simulink model "navigation"  (R2020a)
settings: Solver=VariableStepAuto  StartTime=0.0  StopTime=inf  RelTol=1e-3
model workspace (MAT data in the model file):
  Logfile_Data_Object = robotics.ros.BagSelection
  Logfile_Data_Object.FilePath = '/home/john/github/Thesis-/Control Algorithms/Navigation_Stack/Experiment_6_Plots/2022-08-07-23-07-18.bag'
  Logfile_Data_Object.StartTime = 1659877638.2
  Logfile_Data_Object.EndTime = 1659877673.93
  Logfile_Data_Object.NumMessages = 1808
  Logfile_Data_Object.AvailableTopics = table
  Logfile_Data_Object.AvailableTopics.data{1} = [36; 36; 714; 1022]
  Logfile_Data_Object.AvailableTopics.data{2} = categorical
  Logfile_Data_Object.AvailableTopics.data{2}.categoryNames = {'nav_msgs/Odometry'; 'std_msgs/Float32'; 'std_msgs/Float32MultiArray'}
  Logfile_Data_Object.AvailableTopics.data{2}.codes = [2; 2; 1; 3]
  Logfile_Data_Object.AvailableTopics.data{3}{1} = ''
  Logfile_Data_Object.AvailableTopics.data{3}{2} = ''
  Logfile_Data_Object.AvailableTopics.data{3}{3} = '  uint32 Seq
    |   Time Stamp
    |   char FrameId
    | char ChildFrameId
    | geometry_msgs/PoseWithCovariance Pose
    |   geometry_msgs/Pose Pose
    |     geometry_msgs/Point Position
    |       double X
    |       double Y
    |       double Z
    |     geometry_msgs/Quaternion Orientation
    |       double X
    |       double Y
    |       double Z
    |       double W
    |   double[36] Covariance
    | geometry_msgs/TwistWithCovariance Twist
    |   geometry_msgs/Twist Twist
    |     geometry_msgs/Vector3 Linear
    |       double X
    |       double Y
    |       double Z
    |     geometry_msgs/Vector3 Angular
    |       double X
    |       double Y
    |       double Z
    |   double[36] Covariance
    | '
  Logfile_Data_Object.AvailableTopics.data{3}{4} = '  std_msgs/MultiArrayDimension[] Dim
    |     char Label
    |     uint32 Size
    |     uint32 Stride
    |   uint32 DataOffset
    | single[] Data
    | '
  Logfile_Data_Object.AvailableTopics.ndims = 2
  Logfile_Data_Object.AvailableTopics.nrows = 4
  Logfile_Data_Object.AvailableTopics.rownames = {'/amr/status/current'; '/amr/status/voltage'; '/slamware_ros_sdk_server_node/odom'; '/zlac8015d/encoder'}
  Logfile_Data_Object.AvailableTopics.nvars = 3
  Logfile_Data_Object.AvailableTopics.varnames = {'NumMessages', 'MessageType', 'MessageDefinition'}
  Logfile_Data_Object.AvailableTopics.props.useVariableNamesOriginal = 0
  Logfile_Data_Object.AvailableTopics.props.useDimensionNamesOriginal = 0
  Logfile_Data_Object.AvailableTopics.props.CustomProps = struct()
  Logfile_Data_Object.AvailableTopics.props.VariableCustomProps = struct()
  Logfile_Data_Object.AvailableTopics.props.versionSavedFrom = 4
  Logfile_Data_Object.AvailableTopics.props.minCompatibleVersion = 1
  Logfile_Data_Object.AvailableTopics.props.incompatibilityMsg = ''
  Logfile_Data_Object.AvailableTopics.props.VersionSavedFrom = 4
  Logfile_Data_Object.AvailableTopics.props.Description = ''
  Logfile_Data_Object.AvailableTopics.props.VariableNamesOriginal = {}
  Logfile_Data_Object.AvailableTopics.props.DimensionNames = {'Row', 'Variables'}
  Logfile_Data_Object.AvailableTopics.props.DimensionNamesOriginal = {}
  Logfile_Data_Object.AvailableTopics.props.UserData = []
  Logfile_Data_Object.AvailableTopics.props.VariableDescriptions = {}
  Logfile_Data_Object.AvailableTopics.props.VariableUnits = {}
  Logfile_Data_Object.AvailableTopics.props.VariableContinuity = {}
  Logfile_Data_Object.MessageList = table
  Logfile_Data_Object.MessageList.data{1} = [1659877638.2 1659877638.22 1659877638.24 1659877638.25 1659877638.29 1659877638.29 1659877638.32 1659877638.34 1659877638.35 1659877638.38 1659877638.39 1659877638.41 ... (1808 elements, 1808x1)]
  Logfile_Data_Object.MessageList.data{2} = categorical
  Logfile_Data_Object.MessageList.data{2}.categoryNames = {'/amr/status/current'; '/amr/status/voltage'; '/slamware_ros_sdk_server_node/odom'; '/zlac8015d/encoder'}
  Logfile_Data_Object.MessageList.data{2}.codes = [3 4 3 4 4 3 4 3 4 4 3 4 ... (1808 elements, 1808x1)]
  Logfile_Data_Object.MessageList.data{3} = categorical
  Logfile_Data_Object.MessageList.data{3}.categoryNames = {'std_msgs/Float32'; 'nav_msgs/Odometry'; 'std_msgs/Float32MultiArray'}
  Logfile_Data_Object.MessageList.data{3}.codes = [2 3 2 3 3 2 3 2 3 3 2 3 ... (1808 elements, 1808x1)]
  Logfile_Data_Object.MessageList.data{4} = [7710 10178 10256 11007 11085 11163 11914 11992 12743 12821 12899 13650 ... (1808 elements, 1808x1)]
  Logfile_Data_Object.MessageList.ndims = 2
  Logfile_Data_Object.MessageList.nrows = 1808
  Logfile_Data_Object.MessageList.nvars = 4
  Logfile_Data_Object.MessageList.varnames = {'Time', 'Topic', 'MessageType', 'FileOffset'}
  Logfile_Data_Object.MessageList.props.useVariableNamesOriginal = 0
  Logfile_Data_Object.MessageList.props.useDimensionNamesOriginal = 0
  Logfile_Data_Object.MessageList.props.CustomProps = struct()
  Logfile_Data_Object.MessageList.props.VariableCustomProps = struct()
  Logfile_Data_Object.MessageList.props.versionSavedFrom = 4
  Logfile_Data_Object.MessageList.props.minCompatibleVersion = 1
  Logfile_Data_Object.MessageList.props.incompatibilityMsg = ''
  Logfile_Data_Object.MessageList.props.VersionSavedFrom = 4
  Logfile_Data_Object.MessageList.props.Description = ''
  Logfile_Data_Object.MessageList.props.VariableNamesOriginal = {}
  Logfile_Data_Object.MessageList.props.DimensionNames = {'Row', 'Variables'}
  Logfile_Data_Object.MessageList.props.DimensionNamesOriginal = {}
  Logfile_Data_Object.MessageList.props.UserData = []
  Logfile_Data_Object.MessageList.props.VariableDescriptions = {}
  Logfile_Data_Object.MessageList.props.VariableUnits = {}
  Logfile_Data_Object.MessageList.props.VariableContinuity = {}
  Logfile_Data_Object.TopicTypeMap = containers.Map
  Logfile_Data_Object.TopicTypeMap.serialization.keys = {'/amr/status/current', '/amr/status/voltage', '/slamware_ros_sdk_server_node/odom', '/zlac8015d/encoder'}
  Logfile_Data_Object.TopicTypeMap.serialization.values = {'std_msgs/Float32', 'std_msgs/Float32', 'nav_msgs/Odometry', 'std_msgs/Float32MultiArray'}
  Logfile_Data_Object.TopicTypeMap.serialization.uniformity = 1
  Logfile_Data_Object.TopicTypeMap.serialization.keyType = 'char'
  Logfile_Data_Object.TopicTypeMap.serialization.valueType = 'char'
  Logfile_Data_Object.TopicDefinitionMap = containers.Map
  Logfile_Data_Object.TopicDefinitionMap.serialization.keys = {'/amr/status/current', '/amr/status/voltage', '/slamware_ros_sdk_server_node/odom', '/zlac8015d/encoder'}
  Logfile_Data_Object.TopicDefinitionMap.serialization.values{1} = ''
  Logfile_Data_Object.TopicDefinitionMap.serialization.values{2} = ''
  Logfile_Data_Object.TopicDefinitionMap.serialization.values{3} = '  uint32 Seq
    |   Time Stamp
    |   char FrameId
    | char ChildFrameId
    | geometry_msgs/PoseWithCovariance Pose
    |   geometry_msgs/Pose Pose
    |     geometry_msgs/Point Position
    |       double X
    |       double Y
    |       double Z
    |     geometry_msgs/Quaternion Orientation
    |       double X
    |       double Y
    |       double Z
    |       double W
    |   double[36] Covariance
    | geometry_msgs/TwistWithCovariance Twist
    |   geometry_msgs/Twist Twist
    |     geometry_msgs/Vector3 Linear
    |       double X
    |       double Y
    |       double Z
    |     geometry_msgs/Vector3 Angular
    |       double X
    |       double Y
    |       double Z
    |   double[36] Covariance
    | '
  Logfile_Data_Object.TopicDefinitionMap.serialization.values{4} = '  std_msgs/MultiArrayDimension[] Dim
    |     char Label
    |     uint32 Size
    |     uint32 Stride
    |   uint32 DataOffset
    | single[] Data
    | '
  Logfile_Data_Object.TopicDefinitionMap.serialization.uniformity = 1
  Logfile_Data_Object.TopicDefinitionMap.serialization.keyType = 'char'
  Logfile_Data_Object.TopicDefinitionMap.serialization.valueType = 'char'
  Logfile_Data_Object.Parser = robotics.ros.internal.tf.TransformationTreeParser
  Logfile_Path = '/home/john/github/Thesis-/Control Algorithms/Navigation_Stack/Experiment_6_Plots/2022-08-07-23-07-18.bag'
  Logfile_Playback_Duration = nan
  Logfile_Playback_Offset = nan
values from neighbouring files (symbols this model uses):
  C = [1 0 0 ... (first row only)    [start.m]
  D = [0 0 ... (first row only)    [start.m]
  encoderSampleRate = 10    [start.m]
  firstGoal = [1.5,1.5]    [start.m]
  initialInput = [0; 0]    [start.m]
  initialPose = [0, 0, 0]    [start.m]
  L2RTransform = [cos(L2Rtheta), -sin(L2Rtheta), L2Rx ... (first row only)    [start.m]    (also in test.m = [0.0073926; -0.32076; (3/2)*pi])
  LIVE_MODE = 1    [start.m]
  pose = [0;0;0]    [test.m]
  R = diag(RVar*ones(yNum,1))    [start.m]
  secondGoal = [0.5,0.5]    [start.m]
  timeStep = 0.1    [start.m]
  W2LOTransform = [cos(W2LOtheta), -sin(W2LOtheta), W2LOx ... (first row only)    [start.m]
  W2ORTransform = [cos(W2ORtheta), -sin(W2ORtheta), W2ORx ... (first row only)    [start.m]
  wheelBase = 0.4464    [start.m]
  wheelRadius = 0.1715/2    (= 0.08575)    [start.m]
undefined symbols (not defined in the file or in its folder): Angular, Discrete, goalLoc, startLoc, Time
libraries: robotlib x9, simulink x5, robotmobilelib x3, robotalgslib x3, ctrlSharedLib x1
settings Model: EnablePacing=on  Creator=johni  LastModifiedBy=john

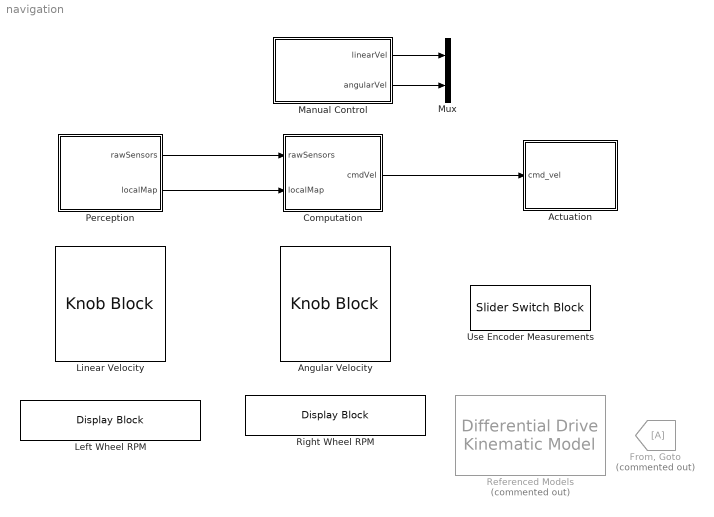
== system navigation ==
  Actuation : Subsystem
  Angular Velocity : KnobBlock  ScaleMin=-1  ScaleMax=1
  Computation : Subsystem
  "From, Goto" : Goto  Commented=on
  Left Wheel RPM : DisplayBlock  LabelPosition=Hide  Format=short  Transparency=1
  Linear Velocity : KnobBlock  ScaleMin=-0.5  ScaleMax=0.5
  Manual Control : Subsystem
  Mux : Mux  Inputs=2
  Perception : Subsystem
  Referenced Models : robotmobilelib/Differential Drive Kinematic Model  Commented=on  VehicleInputs=Wheel Speeds  WheelRadius=0.05  WheelSpeedRange=[-inf inf]  TrackWidth=0.2  InitialState=[0; 0; 0]  SimulateUsing=Interpreted execution
      settings: SourceProductBaseCode=RO
  Right Wheel RPM : DisplayBlock  LabelPosition=Hide  Format=short  Transparency=1
  Use Encoder Measurements : SliderSwitchBlock
      settings: Values={{'Off', 'On'}, [0 1]}
  wires:
  Perception/1(rawSensors) -> Computation/1(rawSensors)
  Perception/2(localMap) -> Computation/2(localMap)
  Manual Control/2(angularVel) -> Mux/2
  Manual Control/1(linearVel) -> Mux/1
  Computation/1(cmdVel) -> Actuation/1(cmd_vel)

== system navigation/Actuation ==
  cmd_vel : Inport
  Actuator : Subsystem
  Demux : Demux  Outputs=2
  Forward Kinematics : Subsystem
  Subsystem : Subsystem  Commented=on
  wires:
  cmd_vel/1 -> Demux/1
  Forward Kinematics/1(leftRpmOut) -> Subsystem/1(leftRPM), Actuator/1(leftRPM)
  Forward Kinematics/2(rightRpmOut) -> Subsystem/2(rightRPM), Actuator/2(rightRPM)
  Demux/2 -> Forward Kinematics/2(w_in)
  Demux/1 -> Forward Kinematics/1(v_in)

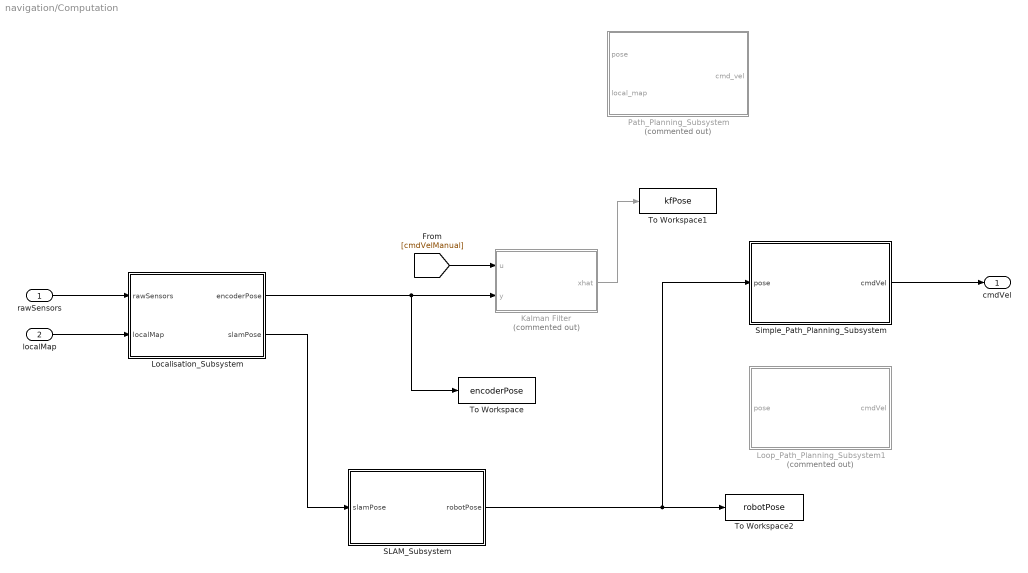
== system navigation/Computation ==
  rawSensors : Inport
  localMap : Inport  Port=2
  Kalman Filter : Subsystem  Commented=on
  Localisation_Subsystem : Subsystem
  Loop_Path_Planning_Subsystem1 : Subsystem  Commented=on
  Path_Planning_Subsystem : Subsystem  Commented=on
  SLAM_Subsystem : Subsystem
  Simple_Path_Planning_Subsystem : Subsystem
  To Workspace : ToWorkspace  VariableName=encoderPose  SaveFormat=Timeseries  SampleTime=-1
  To Workspace1 : ToWorkspace  VariableName=kfPose  SaveFormat=Timeseries  SampleTime=-1
  To Workspace2 : ToWorkspace  VariableName=robotPose  SaveFormat=Timeseries  SampleTime=-1
  cmdVel : Outport
  wires:
  rawSensors/1 -> Localisation_Subsystem/1(rawSensors)
  localMap/1 -> Localisation_Subsystem/2(localMap)
  Localisation_Subsystem/1(encoderPose) -> To Workspace/1, Kalman Filter/2(y)
  SLAM_Subsystem/1(robotPose) -> Simple_Path_Planning_Subsystem/1(pose), To Workspace2/1
  Kalman Filter/1(xhat) -> To Workspace1/1
  [cmdVelManual] -> Kalman Filter/1(u)
  Localisation_Subsystem/2(slamPose) -> SLAM_Subsystem/1(slamPose)
  Simple_Path_Planning_Subsystem/1(cmdVel) -> cmdVel/1

== system navigation/Manual Control ==
  Constant1 : Constant  Value=-0.0004086893464075869
  Constant2 : Constant  Value=0.01208821805826843
  linearVel : Outport
  angularVel : Outport  Port=2
  wires:
  Constant2/1 -> angularVel/1
  Constant1/1 -> linearVel/1

== system navigation/Perception ==
  Encoder_Subsystem : Subsystem
  IMU_Subsystem : Subsystem  Commented=on
  Lidar_Subsystem : Subsystem
  Mux2 : Mux  Inputs=6
  rawSensors : Outport
  localMap : Outport  Port=2
  wires:
  Mux2/1 -> rawSensors/1
  Lidar_Subsystem/3(localMap) -> localMap/1
  IMU_Subsystem/2(linearAcceleration) -> Mux2/4
  IMU_Subsystem/1(angularVelocity) -> Mux2/3
  Lidar_Subsystem/2(slamPose) -> Mux2/6
  Lidar_Subsystem/1(laserScan) -> Mux2/5
  Encoder_Subsystem/2(rightSpeed) -> Mux2/2
  Encoder_Subsystem/1(leftSpeed) -> Mux2/1

== system navigation/Actuation/Actuator ==
  leftRPM : Inport
  rightRPM : Inport  Port=2
  Blank Message : robotlib/Blank Message  messageClass=Message  entityType=geometry_msgs/Twist  messageType=geometry_msgs/Twist  SampleTime=inf
  Bus Assignment : BusAssignment  AssignedSignals=Angular.X,Angular.Y
  Publish : robotlib/Publish  topicSource=Select from ROS network  topic=/zlac8015d/rpm  messageType=geometry_msgs/Twist  messageQueueLength=1
  wires:
  Bus Assignment/1 -> Publish/1
  Blank Message/1 -> Bus Assignment/1
  rightRPM/1 -> Bus Assignment/3
  leftRPM/1 -> Bus Assignment/2

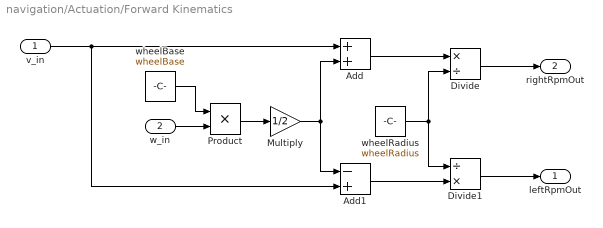
== system navigation/Actuation/Forward Kinematics ==
  v_in : Inport
  w_in : Inport  Port=2
  Add : Sum
  Add1 : Sum  Inputs=-+
  Divide : Product  Inputs=*/
  Divide1 : Product  Inputs=/*
  Multiply : Gain  Gain=1/2
  Product : Product
  wheelBase : Constant  Value=wheelBase
  wheelRadius : Constant  Value=wheelRadius
  leftRpmOut : Outport
  rightRpmOut : Outport  Port=2
  wires:
  v_in/1 -> Add1/2, Add/1
  w_in/1 -> Product/2
  wheelBase/1 -> Product/1
  Product/1 -> Multiply/1
  Multiply/1 -> Add/2, Add1/1
  Add1/1 -> Divide1/2
  Add/1 -> Divide/1
  wheelRadius/1 -> Divide1/1, Divide/2
  Divide1/1 -> leftRpmOut/1
  Divide/1 -> rightRpmOut/1

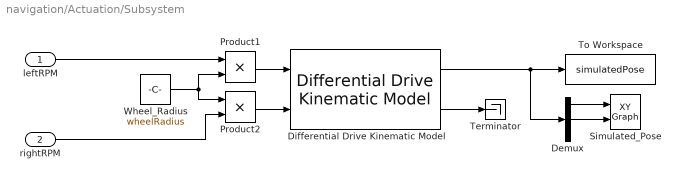
== system navigation/Actuation/Subsystem ==
  leftRPM : Inport
  rightRPM : Inport  Port=2
  Demux : Demux  Outputs=3
  Differential Drive Kinematic Model : robotmobilelib/Differential Drive Kinematic Model  VehicleInputs=Wheel Speeds  WheelRadius=wheelRadius  WheelSpeedRange=[-inf inf]  TrackWidth=wheelBase  InitialState=initialPose  SimulateUsing=Interpreted execution
      settings: SourceProductBaseCode=RO
  Product1 : Product
  Product2 : Product
  Simulated_Pose : simulink/Sinks/XY Graph  xmin=-1.5  xmax=1.5  ymin=-1.5  ymax=1.5  st=-1
  Terminator : Terminator
  To Workspace : ToWorkspace  VariableName=simulatedPose  SaveFormat=Timeseries  SampleTime=-1
  Wheel_Radius : Constant  Value=wheelRadius
  wires:
  Differential Drive Kinematic Model/1 -> Demux/1, To Workspace/1
  Differential Drive Kinematic Model/2 -> Terminator/1
  Demux/2 -> Simulated_Pose/2
  Demux/1 -> Simulated_Pose/1
  Product2/1 -> Differential Drive Kinematic Model/2
  Wheel_Radius/1 -> Product2/1, Product1/2
  leftRPM/1 -> Product1/1
  rightRPM/1 -> Product2/2
  Product1/1 -> Differential Drive Kinematic Model/1

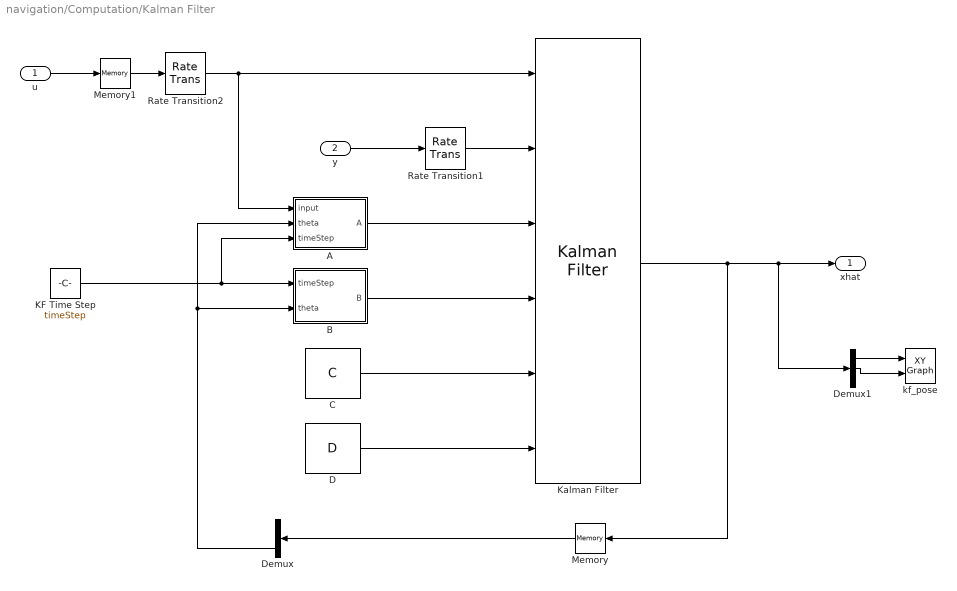
== system navigation/Computation/Kalman Filter ==
  u : Inport
  y : Inport  Port=2
  A : MATLAB Function  TreatAsAtomicUnit=on
  B : MATLAB Function  TreatAsAtomicUnit=on
  C : Constant  Value=C
  D : Constant  Value=D
  Demux : Demux  Outputs=3
  Demux1 : Demux  Outputs=3
  KF Time Step : Constant  Value=timeStep
  Kalman Filter : ctrlSharedLib/Kalman Filter  TimeDomain=Discrete-Time  UseCurrentEstimator=on  ModelSource=Input port  ModelSourceVariable=ss(0.95,1,1,0,1)  A=[1 0 0; 0 1 0; 0 0 1;]  B=[cos(pose(1,3))*timeStep, 0; sin(pose(1,3))*timeStep, 0; 0 timeStep;]  C=[1 0 0; 0 1 0; 0 0 1;]  D=[0,0; 0,0; 0,0;]  NumberOfStates=xNum  NumberOfInputs=uNum  NumberOfOutputs=yNum  InitialEstimateSource=Dialog  X0=initialPose  P0=initialErrorCovariance  UseK=off  UseGH=off  NumberOfProcessNoiseInputs=1  G=1  TimeInvariantG=on  H=0  TimeInvariantH=on  Q=Q  TimeInvariantQ=on  R=R  TimeInvariantR=on  N=0  TimeInvariantN=on  AddInputPort=on  AddEnablePort=off  OutputEstimatedY=off  OutputP=off  Ts=timeStep
  Memory : Memory  InitialCondition=initialPose  InheritSampleTime=on
  Memory1 : Memory  InitialCondition=initialInput  InheritSampleTime=on
  Rate Transition1 : RateTransition  OutPortSampleTime=timeStep
  Rate Transition2 : RateTransition  OutPortSampleTime=timeStep
  kf_pose : simulink/Sinks/XY Graph  xmin=-3  xmax=3  ymin=-3  ymax=3  st=-1
  xhat : Outport
  wires:
  Kalman Filter/1 -> Demux1/1, xhat/1, Memory/1
  u/1 -> Memory1/1
  A/1(A) -> Kalman Filter/3
  C/1 -> Kalman Filter/5
  D/1 -> Kalman Filter/6
  Demux/3 -> A/2(theta), B/2(theta)
  B/1(B) -> Kalman Filter/4
  Memory/1 -> Demux/1
  KF Time Step/1 -> B/1(timeStep), A/3(timeStep)
  y/1 -> Rate Transition1/1
  Rate Transition1/1 -> Kalman Filter/2
  Memory1/1 -> Rate Transition2/1
  Demux1/1 -> kf_pose/1
  Demux1/2 -> kf_pose/2
  Rate Transition2/1 -> A/1(input), Kalman Filter/1

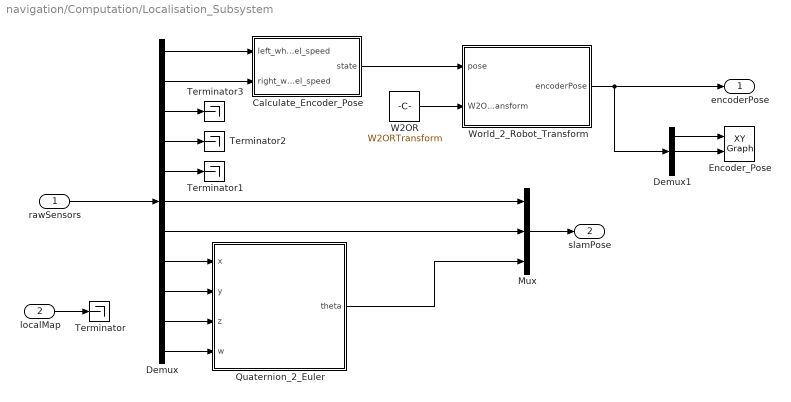
== system navigation/Computation/Localisation_Subsystem ==
  rawSensors : Inport
  localMap : Inport  Port=2
  Calculate_Encoder_Pose : Subsystem
  Demux : Demux  Outputs=11
  Demux1 : Demux  Outputs=3
  Encoder_Pose : simulink/Sinks/XY Graph  xmin=-1.5  xmax=1.5  ymin=-1.5  ymax=1.5  st=-1
  Mux : Mux  Inputs=3
  Quaternion_2_Euler : MATLAB Function  TreatAsAtomicUnit=on
  Terminator{,1..3} (4 alike) : Terminator
  W2OR : Constant  Value=W2ORTransform
  World_2_Robot_Transform : MATLAB Function  TreatAsAtomicUnit=on
  encoderPose : Outport
  slamPose : Outport  Port=2
  wires:
  rawSensors/1 -> Demux/1
  localMap/1 -> Terminator/1
  Demux/1 -> Calculate_Encoder_Pose/1(left_wheel_speed)
  Demux/2 -> Calculate_Encoder_Pose/2(right_wheel_speed)
  Demux/3 -> Terminator3/1
  Demux1/1 -> Encoder_Pose/1
  Demux1/2 -> Encoder_Pose/2
  Demux/4 -> Terminator2/1
  Demux/7 -> Mux/2
  Demux/6 -> Mux/1
  Demux/5 -> Terminator1/1
  Mux/1 -> slamPose/1
  Calculate_Encoder_Pose/1(state) -> World_2_Robot_Transform/1(pose)
  World_2_Robot_Transform/1(encoderPose) -> encoderPose/1, Demux1/1
  W2OR/1 -> World_2_Robot_Transform/2(W2ORTransform)
  Demux/8 -> Quaternion_2_Euler/1(x)
  Demux/9 -> Quaternion_2_Euler/2(y)
  Demux/10 -> Quaternion_2_Euler/3(z)
  Demux/11 -> Quaternion_2_Euler/4(w)
  Quaternion_2_Euler/1(theta) -> Mux/3

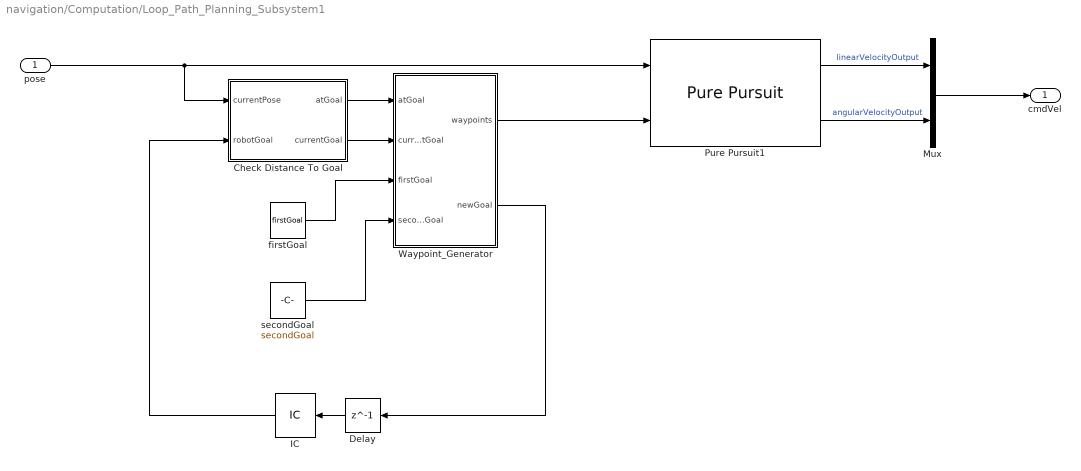
== system navigation/Computation/Loop_Path_Planning_Subsystem1 ==
  pose : Inport
  Check Distance To Goal : Subsystem
  Delay : Delay  DelayLength=1  InitialCondition=0
  IC : InitialCondition  Value=firstGoal
  Mux : Mux  Inputs=2
  Pure Pursuit1 : robotalgslib/Pure Pursuit  DesiredLinearVelocity=0.5  MaxAngularVelocity=1  LookaheadDistance=0.1  TargetDirPort=off  SimulateUsing=Code generation
  Waypoint_Generator : MATLAB Function  TreatAsAtomicUnit=on
  firstGoal : Constant  Value=firstGoal  VectorParams1D=off
  secondGoal : Constant  Value=secondGoal  VectorParams1D=off
  cmdVel : Outport
  wires:
  Mux/1 -> cmdVel/1
  pose/1 -> Check Distance To Goal/1(currentPose), Pure Pursuit1/1
  Pure Pursuit1/2 -> Mux/2  "angularVelocityOutput"
  Pure Pursuit1/1 -> Mux/1  "linearVelocityOutput"
  Check Distance To Goal/1(atGoal) -> Waypoint_Generator/1(atGoal)
  Check Distance To Goal/2(currentGoal) -> Waypoint_Generator/2(currentGoal)
  Waypoint_Generator/1(waypoints) -> Pure Pursuit1/2
  firstGoal/1 -> Waypoint_Generator/3(firstGoal)
  secondGoal/1 -> Waypoint_Generator/4(secondGoal)
  Waypoint_Generator/2(newGoal) -> Delay/1
  Delay/1 -> IC/1
  IC/1 -> Check Distance To Goal/2(robotGoal)

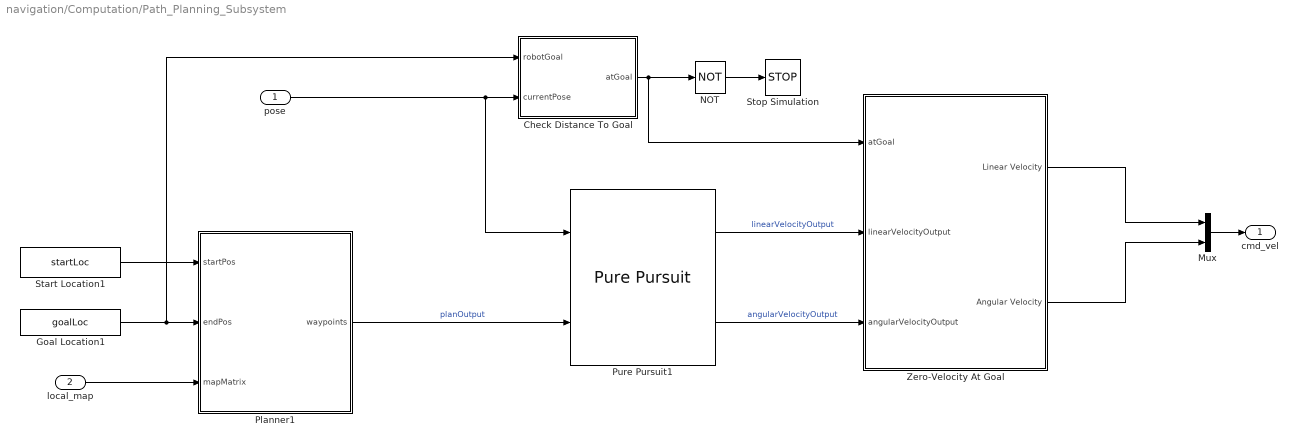
== system navigation/Computation/Path_Planning_Subsystem ==
  pose : Inport
  local_map : Inport  Port=2
  Check Distance To Goal : Subsystem
  Goal Location1 : Constant  Value=goalLoc
  Mux : Mux  Inputs=2
  NOT : Logic  Operator=NOT  IconShape=distinctive  AllPortsSameDT=off  OutDataTypeStr=boolean
  Planner1 : MATLAB Function  TreatAsAtomicUnit=on
  Pure Pursuit1 : robotalgslib/Pure Pursuit  DesiredLinearVelocity=0.1  MaxAngularVelocity=1.0  LookaheadDistance=0.5  TargetDirPort=off  SimulateUsing=Code generation
  Start Location1 : Constant  Value=startLoc
  Stop Simulation : Stop
  Zero-Velocity At Goal : Subsystem
  cmd_vel : Outport
  wires:
  local_map/1 -> Planner1/3(mapMatrix)
  Pure Pursuit1/2 -> Zero-Velocity At Goal/3(angularVelocityOutput)  "angularVelocityOutput"
  Pure Pursuit1/1 -> Zero-Velocity At Goal/2(linearVelocityOutput)  "linearVelocityOutput"
  Planner1/1(waypoints) -> Pure Pursuit1/2  "planOutput"
  NOT/1 -> Stop Simulation/1
  Start Location1/1 -> Planner1/1(startPos)
  Check Distance To Goal/1(atGoal) -> Zero-Velocity At Goal/1(atGoal), NOT/1
  Goal Location1/1 -> Check Distance To Goal/1(robotGoal), Planner1/2(endPos)
  pose/1 -> Pure Pursuit1/1, Check Distance To Goal/2(currentPose)
  Mux/1 -> cmd_vel/1
  Zero-Velocity At Goal/1(Linear Velocity) -> Mux/1
  Zero-Velocity At Goal/2(Angular Velocity) -> Mux/2

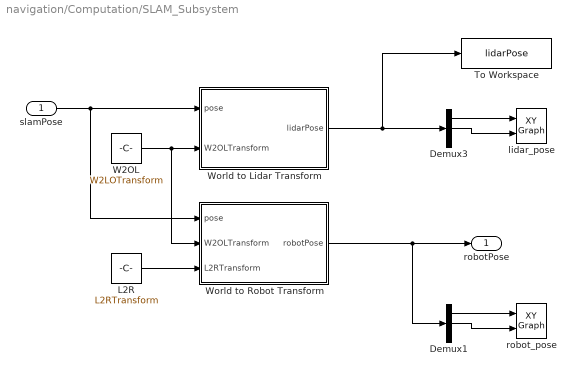
== system navigation/Computation/SLAM_Subsystem ==
  slamPose : Inport
  Demux1 : Demux  Outputs=3
  Demux3 : Demux  Outputs=3
  L2R : Constant  Value=L2RTransform
  To Workspace : ToWorkspace  VariableName=lidarPose  SaveFormat=Timeseries  SampleTime=-1
  W2OL : Constant  Value=W2LOTransform
  World to Lidar Transform : MATLAB Function  TreatAsAtomicUnit=on
  World to Robot Transform : MATLAB Function  TreatAsAtomicUnit=on
  lidar_pose : simulink/Sinks/XY Graph  xmin=0  xmax=3  ymin=0  ymax=3  st=-1
  robot_pose : simulink/Sinks/XY Graph  xmin=0  xmax=3  ymin=0  ymax=3  st=-1
  robotPose : Outport
  wires:
  Demux1/2 -> robot_pose/2
  Demux1/1 -> robot_pose/1
  slamPose/1 -> World to Robot Transform/1(pose), World to Lidar Transform/1(pose)
  World to Robot Transform/1(robotPose) -> robotPose/1, Demux1/1
  World to Lidar Transform/1(lidarPose) -> To Workspace/1, Demux3/1
  Demux3/1 -> lidar_pose/1
  Demux3/2 -> lidar_pose/2
  L2R/1 -> World to Robot Transform/3(L2RTransform)
  W2OL/1 -> World to Lidar Transform/2(W2OLTransform), World to Robot Transform/2(W2OLTransform)

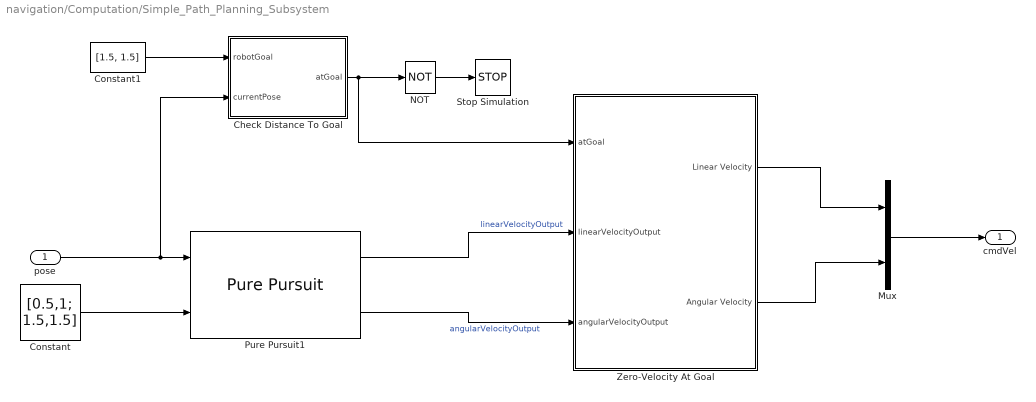
== system navigation/Computation/Simple_Path_Planning_Subsystem ==
  pose : Inport
  Check Distance To Goal : Subsystem
  Constant : Constant  Value=[0.5,1; 1.5,1.5]
  Constant1 : Constant  Value=[1.5, 1.5]
  Mux : Mux  Inputs=2
  NOT : Logic  Operator=NOT  IconShape=distinctive  AllPortsSameDT=off  OutDataTypeStr=boolean
  Pure Pursuit1 : robotalgslib/Pure Pursuit  DesiredLinearVelocity=0.5  MaxAngularVelocity=1  LookaheadDistance=0.1  TargetDirPort=off  SimulateUsing=Code generation
  Stop Simulation : Stop
  Zero-Velocity At Goal : Subsystem
  cmdVel : Outport
  wires:
  Mux/1 -> cmdVel/1
  pose/1 -> Check Distance To Goal/2(currentPose), Pure Pursuit1/1
  Constant/1 -> Pure Pursuit1/2
  Check Distance To Goal/1(atGoal) -> Zero-Velocity At Goal/1(atGoal), NOT/1
  NOT/1 -> Stop Simulation/1
  Pure Pursuit1/1 -> Zero-Velocity At Goal/2(linearVelocityOutput)  "linearVelocityOutput"
  Pure Pursuit1/2 -> Zero-Velocity At Goal/3(angularVelocityOutput)  "angularVelocityOutput"
  Zero-Velocity At Goal/2(Angular Velocity) -> Mux/2
  Zero-Velocity At Goal/1(Linear Velocity) -> Mux/1
  Constant1/1 -> Check Distance To Goal/1(robotGoal)

== system navigation/Perception/Encoder_Subsystem ==
  LIVE_MODE : Constant  Value=LIVE_MODE
  Parse_Encoder : Subsystem
  Read Data : robotlib/Read Data  topic=/zlac8015d/encoder  sampleTime=-1  logfileType=rosbag  modelName=navigation  msgType=std_msgs/Float32MultiArray
      settings: SourceProductBaseCode=RR
  Subscribe : robotlib/Subscribe  topicSource=Select from ROS network  topic=/zlac8015d/encoder  messageType=std_msgs/Float32MultiArray  sampleTime=encoderSampleRate  messageQueueLength=1
  Switch : Switch  Threshold=1
  leftSpeed : Outport
  rightSpeed : Outport  Port=2
  wires:
  Parse_Encoder/1(leftSpeed) -> leftSpeed/1
  Parse_Encoder/2(rightSpeed) -> rightSpeed/1
  Switch/1 -> Parse_Encoder/1(Msg)
  LIVE_MODE/1 -> Switch/2
  Read Data/2 -> Switch/3
  Subscribe/2 -> Switch/1

== system navigation/Perception/IMU_Subsystem ==
  Bus Selector : BusSelector  OutputSignals=AngularVelocity.Z,LinearAcceleration.X
  Subscribe : robotlib/Subscribe  topicSource=Select from ROS network  topic=/imu/data  messageType=sensor_msgs/Imu  sampleTime=-1  messageQueueLength=1
  angularVelocity : Outport
  linearAcceleration : Outport  Port=2
  wires:
  Subscribe/2 -> Bus Selector/1
  Bus Selector/1 -> angularVelocity/1  "<Z>"
  Bus Selector/2 -> linearAcceleration/1  "<X>"

== system navigation/Perception/Lidar_Subsystem ==
  Bus Selector : BusSelector  Commented=on  OutputSignals=Data
  Bus Selector1 : BusSelector  Commented=on  OutputSignals=AngleIncrement,TimeIncrement,Ranges
  SLAM_Pose_Subsystem : Subsystem
  Subscribe1 : robotlib/Subscribe  Commented=on  topicSource=Select from ROS network  topic=/slamware_ros_sdk_server_node/map  messageType=nav_msgs/OccupancyGrid  sampleTime=-1  messageQueueLength=1
  Subscribe2 : robotlib/Subscribe  Commented=on  topicSource=Select from ROS network  topic=/slamware_ros_sdk_server_node/scan  messageType=sensor_msgs/LaserScan  sampleTime=-1  messageQueueLength=1
  laserScan : Outport
  slamPose : Outport  Port=2
  localMap : Outport  Port=3
  wires:
  Subscribe2/2 -> Bus Selector1/1
  Bus Selector/1 -> localMap/1  "<Data>"
  Subscribe1/2 -> Bus Selector/1
  SLAM_Pose_Subsystem/1(slamPose) -> slamPose/1

== system navigation/Computation/Localisation_Subsystem/Calculate_Encoder_Pose ==
  left_wheel_speed : Inport
  right_wheel_speed : Inport  Port=2
  Differential Drive Kinematic Model : robotmobilelib/Differential Drive Kinematic Model  VehicleInputs=Wheel Speeds  WheelRadius=wheelRadius  WheelSpeedRange=[-inf inf]  TrackWidth=wheelBase  InitialState=initialPose  SimulateUsing=Interpreted execution
      settings: SourceProductBaseCode=RO
  Terminator : Terminator
  state : Outport
  wires:
  Differential Drive Kinematic Model/2 -> Terminator/1
  Differential Drive Kinematic Model/1 -> state/1
  right_wheel_speed/1 -> Differential Drive Kinematic Model/2
  left_wheel_speed/1 -> Differential Drive Kinematic Model/1

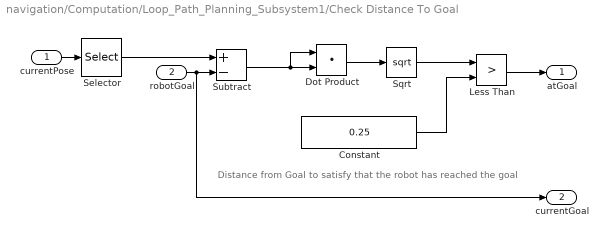
== system navigation/Computation/Loop_Path_Planning_Subsystem1/Check Distance To Goal ==
  note: Distance from Goal to satisfy that the robot has reached the goal
  currentPose : Inport
  robotGoal : Inport  Port=2
  Constant : Constant  Value=0.25
  Dot Product : DotProduct  InputSameDT=on  OutDataTypeStr=Inherit: Inherit via internal rule
  Less Than : RelationalOperator  Operator=>  OutDataTypeStr=boolean  RndMeth=Simplest
  Selector : Selector  InputPortWidth=3  IndexOptions=Index vector (dialog)  Indices=[1 2]  OutputSizes=1
  Sqrt : Sqrt  SaturateOnIntegerOverflow=on
  Subtract : Sum  Inputs=+-
  atGoal : Outport
  currentGoal : Outport  Port=2
  wires:
  robotGoal/1 -> currentGoal/1, Subtract/2
  Dot Product/1 -> Sqrt/1
  Constant/1 -> Less Than/2
  currentPose/1 -> Selector/1
  Less Than/1 -> atGoal/1
  Sqrt/1 -> Less Than/1
  Subtract/1 -> Dot Product/1, Dot Product/2
  Selector/1 -> Subtract/1

== system navigation/Computation/Path_Planning_Subsystem/Check Distance To Goal ==
  note: Distance from Goal to satisfy that the robot has reached the goal
  robotGoal : Inport
  currentPose : Inport  Port=2
  Constant : Constant  Value=0.25
  Dot Product : DotProduct  InputSameDT=on  OutDataTypeStr=Inherit: Inherit via internal rule
  Less Than : RelationalOperator  Operator=>  OutDataTypeStr=boolean  RndMeth=Simplest
  Selector : Selector  InputPortWidth=3  IndexOptions=Index vector (dialog)  Indices=[1 2]  OutputSizes=1
  Sqrt : Sqrt  SaturateOnIntegerOverflow=on
  Subtract : Sum  Inputs=+-
  atGoal : Outport
  wires:
  robotGoal/1 -> Subtract/2
  Dot Product/1 -> Sqrt/1
  Constant/1 -> Less Than/2
  currentPose/1 -> Selector/1
  Less Than/1 -> atGoal/1
  Sqrt/1 -> Less Than/1
  Subtract/1 -> Dot Product/1, Dot Product/2
  Selector/1 -> Subtract/1

== system navigation/Computation/Path_Planning_Subsystem/Zero-Velocity At Goal ==
  atGoal : Inport
  linearVelocityOutput : Inport  Port=2
  angularVelocityOutput : Inport  Port=3
  Product : Product
  Product1 : Product
  Linear Velocity : Outport  OutDataTypeStr=double
  Angular Velocity : Outport  Port=2  OutDataTypeStr=double
  wires:
  atGoal/1 -> Product1/1, Product/1
  angularVelocityOutput/1 -> Product1/2
  linearVelocityOutput/1 -> Product/2
  Product/1 -> Linear Velocity/1
  Product1/1 -> Angular Velocity/1

== system navigation/Computation/Simple_Path_Planning_Subsystem/Check Distance To Goal ==
  note: Distance from Goal to satisfy that the robot has reached the goal
  robotGoal : Inport
  currentPose : Inport  Port=2
  Constant : Constant  Value=0.25
  Dot Product : DotProduct  InputSameDT=on  OutDataTypeStr=Inherit: Inherit via internal rule
  Less Than : RelationalOperator  Operator=>  OutDataTypeStr=boolean  RndMeth=Simplest
  Selector : Selector  InputPortWidth=3  IndexOptions=Index vector (dialog)  Indices=[1 2]  OutputSizes=1
  Sqrt : Sqrt  SaturateOnIntegerOverflow=on
  Subtract : Sum  Inputs=+-
  atGoal : Outport
  wires:
  robotGoal/1 -> Subtract/2
  Dot Product/1 -> Sqrt/1
  Constant/1 -> Less Than/2
  currentPose/1 -> Selector/1
  Less Than/1 -> atGoal/1
  Sqrt/1 -> Less Than/1
  Subtract/1 -> Dot Product/1, Dot Product/2
  Selector/1 -> Subtract/1

== system navigation/Computation/Simple_Path_Planning_Subsystem/Zero-Velocity At Goal ==
  atGoal : Inport
  linearVelocityOutput : Inport  Port=2
  angularVelocityOutput : Inport  Port=3
  Product : Product
  Product1 : Product
  Linear Velocity : Outport  OutDataTypeStr=double
  Angular Velocity : Outport  Port=2  OutDataTypeStr=double
  wires:
  atGoal/1 -> Product1/1, Product/1
  angularVelocityOutput/1 -> Product1/2
  linearVelocityOutput/1 -> Product/2
  Product/1 -> Linear Velocity/1
  Product1/1 -> Angular Velocity/1

== system navigation/Perception/Encoder_Subsystem/Parse_Encoder ==
  Msg : Inport
  Bus Selector : BusSelector  OutputSignals=Data
  Inverse_Kinematics : Subsystem
  Parse_Encoder : MATLAB Function  TreatAsAtomicUnit=on
  leftSpeed : Outport
  rightSpeed : Outport  Port=2
  wires:
  Inverse_Kinematics/2(rightSpeed) -> rightSpeed/1
  Msg/1 -> Bus Selector/1
  Inverse_Kinematics/1(leftSpeed) -> leftSpeed/1
  Bus Selector/1 -> Parse_Encoder/1(msg)  "<Data>"
  Parse_Encoder/1(y) -> Inverse_Kinematics/1(rawEncoder)

== system navigation/Perception/Lidar_Subsystem/SLAM_Pose_Subsystem ==
  LIVE_STATE : Constant  Value=LIVE_MODE
  Pose_Parser : Subsystem
  Read Data : robotlib/Read Data  topic=/slamware_ros_sdk_server_node/odom  sampleTime=-1  logfileType=rosbag  modelName=navigation  msgType=nav_msgs/Odometry
      settings: SourceProductBaseCode=RR
  Subscribe3 : robotlib/Subscribe  topicSource=Select from ROS network  topic=/slamware_ros_sdk_server_node/odom  messageType=nav_msgs/Odometry  sampleTime=-1  messageQueueLength=1
  Switch : Switch  Threshold=1
  slamPose : Outport
  wires:
  Read Data/2 -> Switch/3
  LIVE_STATE/1 -> Switch/2
  Subscribe3/2 -> Switch/1
  Switch/1 -> Pose_Parser/1(msg)
  Pose_Parser/1(slamPose) -> slamPose/1

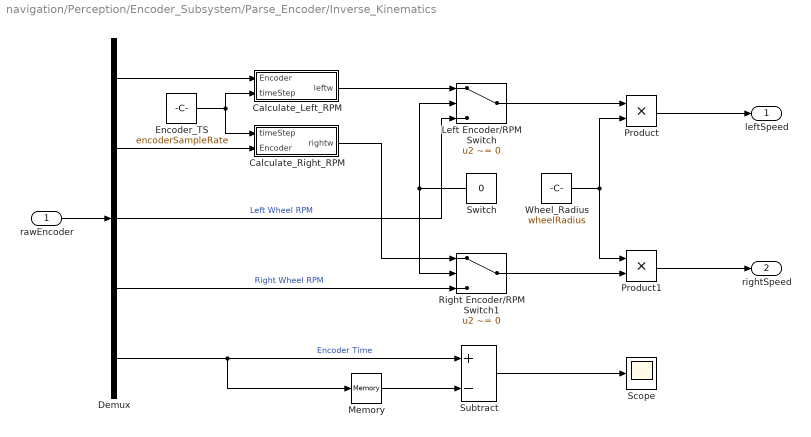
== system navigation/Perception/Encoder_Subsystem/Parse_Encoder/Inverse_Kinematics ==
  rawEncoder : Inport
  Calculate_Left_RPM : Subsystem
  Calculate_Right_RPM : Subsystem
  Demux : Demux  Outputs=5
  Encoder_TS : Constant  Value=encoderSampleRate
  Left Encoder/RPM Switch : Switch  Criteria=u2 ~= 0
  Memory : Memory
  Product : Product
  Product1 : Product
  Right Encoder/RPM Switch1 : Switch  Criteria=u2 ~= 0
  Scope : Scope
  Subtract : Sum  Inputs=+-
  Switch : Constant  Value=0
  Wheel_Radius : Constant  Value=wheelRadius
  leftSpeed : Outport
  rightSpeed : Outport  Port=2
  wires:
  Calculate_Right_RPM/1(rightw) -> Right Encoder/RPM Switch1/1
  Demux/2 -> Calculate_Right_RPM/2(Encoder)
  Switch/1 -> Left Encoder/RPM Switch/2, Right Encoder/RPM Switch1/2
  Demux/1 -> Calculate_Left_RPM/1(Encoder)
  Demux/3 -> Left Encoder/RPM Switch/3  "Left Wheel RPM"
  Demux/4 -> Right Encoder/RPM Switch1/3  "Right Wheel RPM"
  Calculate_Left_RPM/1(leftw) -> Left Encoder/RPM Switch/1
  rawEncoder/1 -> Demux/1
  Encoder_TS/1 -> Calculate_Right_RPM/1(timeStep), Calculate_Left_RPM/2(timeStep)
  Right Encoder/RPM Switch1/1 -> Product1/2
  Wheel_Radius/1 -> Product1/1, Product/2
  Product/1 -> leftSpeed/1
  Product1/1 -> rightSpeed/1
  Left Encoder/RPM Switch/1 -> Product/1
  Demux/5 -> Memory/1, Subtract/1  "Encoder Time"
  Memory/1 -> Subtract/2
  Subtract/1 -> Scope/1

== system navigation/Perception/Lidar_Subsystem/SLAM_Pose_Subsystem/Pose_Parser ==
  msg : Inport
  Bus Selector2 : BusSelector  OutputSignals=Pose.Pose.Position.X,Pose.Pose.Position.Y,Pose.Pose.Orientation.X,Pose.Pose.Orientation.Y,Pose.Pose.Orientation.Z,Pose.Pose.Orientation.W
  Mux : Mux  Inputs=6
  slamPose : Outport
  wires:
  msg/1 -> Bus Selector2/1
  Mux/1 -> slamPose/1
  Bus Selector2/1 -> Mux/1  "<X>"
  Bus Selector2/2 -> Mux/2  "<Y>"
  Bus Selector2/3 -> Mux/3  "<X>"
  Bus Selector2/4 -> Mux/4  "<Y>"
  Bus Selector2/5 -> Mux/5  "<Z>"
  Bus Selector2/6 -> Mux/6  "<W>"

== system navigation/Perception/Encoder_Subsystem/Parse_Encoder/Inverse_Kinematics/Calculate_Left_RPM ==
  Encoder : Inport
  timeStep : Inport  Port=2
  Add : Sum  Inputs=+-
  Divide : Product  Inputs=*/
  Gain : Gain  Gain=600
  Memory : Memory
  leftw : Outport
  wires:
  Encoder/1 -> Memory/1, Add/1
  Memory/1 -> Add/2
  timeStep/1 -> Divide/2
  Divide/1 -> leftw/1
  Add/1 -> Gain/1
  Gain/1 -> Divide/1

== system navigation/Perception/Encoder_Subsystem/Parse_Encoder/Inverse_Kinematics/Calculate_Right_RPM ==
  timeStep : Inport
  Encoder : Inport  Port=2
  Add : Sum  Inputs=+-
  Divide : Product  Inputs=*/
  Gain : Gain  Gain=600
  Memory : Memory
  rightw : Outport
  wires:
  Encoder/1 -> Memory/1, Add/1
  Memory/1 -> Add/2
  timeStep/1 -> Divide/2
  Divide/1 -> rightw/1
  Add/1 -> Gain/1
  Gain/1 -> Divide/1

== matlab function navigation/Computation/Kalman Filter/B ==
  data: timeStep input; theta input; B output
function B = fcn(timeStep, theta)
    
    BMatrix = [cos(theta)*timeStep, 0; 
               sin(theta)*timeStep, 0; 
               0, timeStep]; 

B = BMatrix;

== matlab function navigation/Perception/Encoder_Subsystem/Parse_Encoder/Parse_Encoder ==
  data: msg input; y output
function y = fcn(msg)
    
    % Parse Message 
    encoderLeft = msg(1,1); 
    encoderRight = msg(2,1); 
    rpmLeft = msg(3,1); 
    rpmRight = msg(4,1); 
    encoderTime = msg(5,1); 
    
y = [encoderLeft; encoderRight; rpmLeft; rpmRight; encoderTime];

== matlab function navigation/Computation/Kalman Filter/A ==
  data: A output; input input; theta input; timeStep input
function A = fcn(input, theta, timeStep)
    
    v = input(1,1); 

    AMatrix = [1, 0, v*sin(theta)*timeStep; 
               0, 1, v*cos(theta)*timeStep;
               0, 0, 1];
A = AMatrix;

== matlab function navigation/Computation/SLAM_Subsystem/World to Robot Transform ==
  data: pose input; robotPose output; W2OLTransform input; L2RTransform input
function robotPose = fcn(pose, W2OLTransform, L2RTransform)
    
    % O2L Transform 
    OL2LTransform = [cos(pose(3,1)), -sin(pose(3,1)), pose(1,1);
                    sin(pose(3,1)), cos(pose(3,1)), pose(2,1);
                    0,              0,              1];

    % Calculate World to Robot
    W2RTransform = W2OLTransform*OL2LTransform*L2RTransform; 
    

    % Extract relevant information
robotPose = [W2RTransform(1,3); W2RTransform(2,3); acos(W2RTransform(1,1))];

== matlab function navigation/Computation/SLAM_Subsystem/World to Lidar Transform ==
  data: pose input; lidarPose output; W2OLTransform input
function lidarPose = fcn(pose, W2OLTransform)
    
    LVector = [pose(1,1); pose(2,1); 1];
    
    newLVector = W2OLTransform*LVector; 
    
lidarPose = [newLVector(1,1); newLVector(2,1); (3/2)*pi - pose(3,1)];

== matlab function navigation/Computation/Path_Planning_Subsystem/Planner1 ==
  settings: updateMethod=DISCRETE
  data: startPos input size=[1 2]; endPos input size=[1 2]; waypoints output size=[100 2]; mapMatrix input
function waypoints = planning(startPos, endPos, mapMatrix)

persistent waypointsInternal
persistent prevStartPos
persistent prevEndPos

% Set constant parameters
maxNumNodes = 100;

% Initialize persistent variables that are used downstream
if isempty(prevStartPos)
    prevStartPos = startPos;
end

if isempty(prevEndPos)
    prevEndPos = endPos;
end

isNewPath = (~isequal(prevStartPos, startPos) || ~isequal(prevEndPos, endPos));

if isempty(waypointsInternal) || isNewPath
    % Two conditions in which waypoints must be set: they are not yet
    % initialized, or they are initialized, but the current start and end
    % do not match those used to generate the previous set of waypoints
    [waypointsInternal] = planPath(mapMatrix, maxNumNodes, startPos, endPos);
end

% Update the outputs
waypoints = waypointsInternal;

% Update the persistent variables that indicate previous state
prevStartPos = startPos;
prevEndPos = endPos;

%% Helper Function

function wayPoints = planPath(mapMatrix, maxNodes, startPos, endPos)
    
    % Create a probabilistic roadmap
    map = binaryOccupancyMap(mapMatrix);
    prm = mobileRobotPRM(map, maxNodes);
    
    % Find a path between two points
    xy = findpath(prm, startPos, endPos);
    wayPoints = repmat(endPos, maxNodes, 1);
    
    % Number of nodes that are actually used
    numNodes = length(xy);
    wayPoints(1:numNodes,:) = xy;    

end

end

== matlab function navigation/Computation/Localisation_Subsystem/World_2_Robot_Transform ==
  data: pose input; encoderPose output; W2ORTransform input
function encoderPose = fcn(pose, W2ORTransform)
    
    Vector = [pose(1,1); pose(2,1); 1];
    
    newVector = W2ORTransform*Vector; 
    
encoderPose = [newVector(1,1); newVector(2,1); (3/2)*pi - pose(3,1)];

== matlab function navigation/Computation/Localisation_Subsystem/Quaternion_2_Euler ==
  data: x input; theta output; y input; z input; w input
function theta = fcn(x, y, z, w)

    euler = quat2eul([x, y, z, w]); 
    
theta = euler(1,3);

== matlab function navigation/Computation/Loop_Path_Planning_Subsystem1/Waypoint_Generator ==
  data: waypoints output; atGoal input; newGoal output; currentGoal input; firstGoal input; secondGoal input
function [waypoints, newGoal] = fcn(atGoal, currentGoal, firstGoal, secondGoal)

    % Initial condition
    waypoints = [0.5, 1.5; firstGoal];
    newGoal = firstGoal; 
    
    % Check if not
    if isequal(currentGoal,secondGoal)
        waypoints = [1.5, 0.5; secondGoal]; 
        newGoal = secondGoal; 
    end

    % Check current goals 
    if atGoal == 0 && isequal(currentGoal,firstGoal)
        
        newGoal = secondGoal; 
        waypoints = [1.5, 0.5; secondGoal]; 
        
    elseif atGoal == 0 && isequal(currentGoal,secondGoal)
        
        newGoal = firstGoal; 
        waypoints = [0.5, 1.5; firstGoal]; 
        
    end
